simulink model "computed_torque_control"  (R2024b)
settings: Solver=VariableStepAuto  StartTime=0.0  StopTime=20  RelTol=1e-3
values from neighbouring files (symbols this model uses):
  Kp = diag(Kp_degerleri)    [robot_control.m]
  Kv = diag(Kv_degerleri)    [robot_control.m]
settings Model: Creator=burak  LastModifiedBy=burak

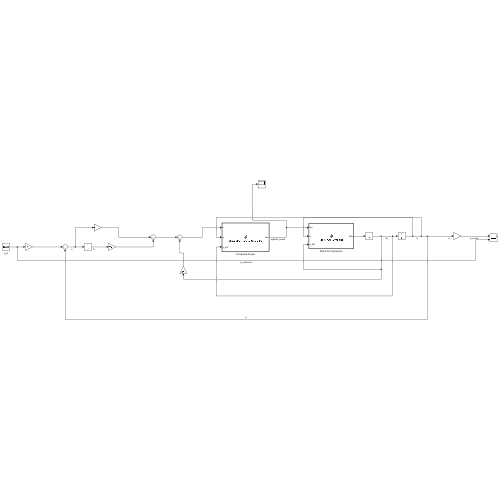
[thumbnail: Simulink's stored preview of the top-level diagram]
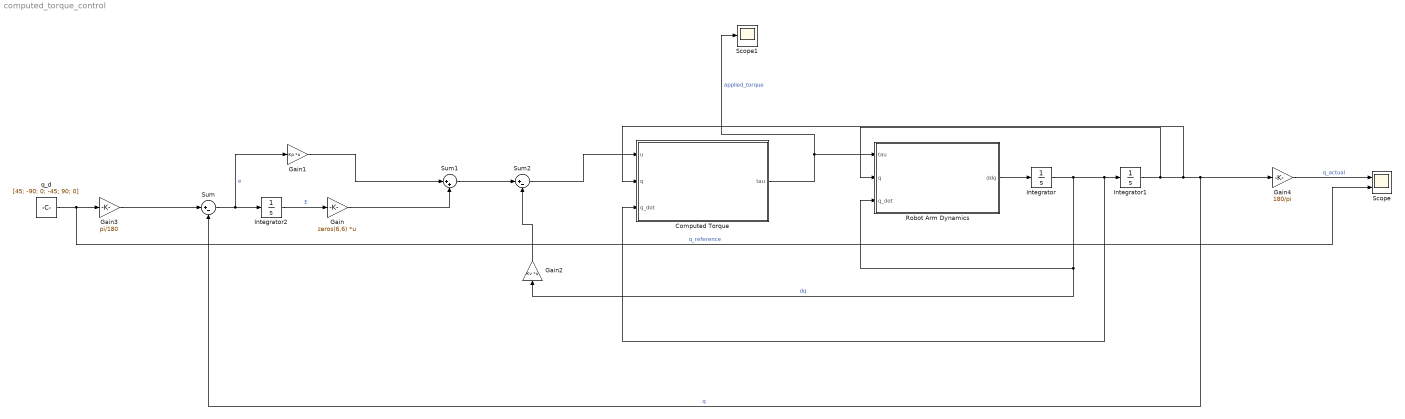
== system computed_torque_control ==
  Computed Torque : MATLAB Function  TreatAsAtomicUnit=on
  Gain : Gain  Gain=zeros(6,6)  Multiplication=Matrix(K*u)
  Gain1 : Gain  Gain=Kp  Multiplication=Matrix(K*u)
  Gain2 : Gain  Gain=Kv  Multiplication=Matrix(K*u)
  Gain3 : Gain  Gain=pi/180
  Gain4 : Gain  Gain=180/pi
  Integrator : Integrator  InitialCondition=zeros(6,1)
  Integrator1 : Integrator  InitialCondition=zeros(6,1)
  Integrator2 : Integrator  InitialCondition=zeros(6,1)
  Robot Arm Dynamics : MATLAB Function  TreatAsAtomicUnit=on
  Scope : Scope  NumInputPorts=2
  Scope1 : Scope
  Sum : Sum  Inputs=|+-
  Sum1 : Sum  Inputs=|++
  Sum2 : Sum  Inputs=|+-
  q_d : Constant  Value=[45; -90; 0; -45; 90; 0]
  wires:
  Robot Arm Dynamics/1(ddq) -> Integrator/1
  Integrator/1 -> Gain2/1, Robot Arm Dynamics/3(q_dot), Computed Torque/3(q_dot), Integrator1/1  "dq"
  Integrator1/1 -> Robot Arm Dynamics/2(q), Computed Torque/2(q), Sum/2, Gain4/1  "q"
  Sum/1 -> Gain1/1, Integrator2/1  "e"
  Integrator2/1 -> Gain/1  "E"
  Gain/1 -> Sum1/2
  Gain1/1 -> Sum1/1
  Computed Torque/1(tau) -> Scope1/1, Robot Arm Dynamics/1(tau)  "applied_torque"
  Sum1/1 -> Sum2/1
  Gain2/1 -> Sum2/2
  Sum2/1 -> Computed Torque/1(u)
  q_d/1 -> Scope/2, Gain3/1  "q_reference"
  Gain3/1 -> Sum/1
  Gain4/1 -> Scope/1  "q_actual"

== matlab function computed_torque_control/Robot Arm Dynamics ==
  data: tau input; ddq output; q input; q_dot input
function ddq = Robot_Arm_Dynamics(tau, q, q_dot)
    D_num = calc_D(q);
    C_num = calc_C(q, q_dot);
    g_num = calc_g(q);
    ddq = D_num \ (tau - C_num * q_dot - g_num);
    
end

== matlab function computed_torque_control/Computed Torque ==
  data: u input; tau output; q input; q_dot input
function tau = Computed_Torque_Controller(u, q, q_dot)
    D_num = calc_D(q);
    C_num = calc_C(q, q_dot);
    g_num = calc_g(q);
    tau = D_num * u + C_num * q_dot + g_num;
    
end
